simulink model "General_MG"  (R2024a)
settings: Solver=VariableStepAuto  StartTime=0.0  StopTime=10.0  RelTol=1e-3
values from neighbouring files (symbols this model uses):
  BarC = [Barc_11, Barc_12, Barc_13, Barc_14 ... (first row only)    [Global_Controller_Synthesis.m]    (also in globalControlDesign-Mohammad’s Laptop.m = zeros(numOfDGs * 3, numOfLines); globalControlDesign.m = zeros(numOfDGs * 3, numOfLines))
  C = [c_11,c_12,c_13,c_14 ... (first row only)    [Global_Controller_Synthesis.m]    (also in centralizedCodesignFeasibility.m = [statusL-ones(numOfDGs,1); statusG-1]; globalControlDesign-Mohammad’s Laptop.m = zeros(numOfLines, numOfDGs * 3); globalControlDesign.m = zeros(numOfLines, numOfDGs * 3))
  DG = cell(1, numOfDGs)    [evaluateDesigns.m]
  H = blkdiag(H, H_i)    [globalControlDesign-Mohammad’s Laptop.m]    (also in globalControlDesign.m)
  K = cell(1, numDGs)    [Centralized_Controller_For_DG.m]    (also in Centralized_Controller_For_DG_with_Constraints.m; ComputePassivityForDGs.m = sdpvar(1, 3, 'full'); GetPassivityForDGs.m = sdpvar(1, 3, 'full'); Global_Controller_Synthesis.m = cell(N, N))
  Line = cell(1, numOfLines)    [evaluateDesigns.m]
  numOfDGs = size(B_il,1)    [OptimizeMGparameters.m]    (also in OptimizepValsMethod1.m; centralizedCodesign.m; centralizedCodesignFeasibility.m; centralizedLocalControlDesign-Mohammad’s Laptop.m)
  numOfLines = size(B_il,2)    [OptimizeMGparameters.m]    (also in OptimizepValsMethod1.m; centralizedCodesign.m; centralizedCodesignFeasibility.m; centralizedLocalControlDesign-Mohammad’s Laptop.m)
  V_ref = 48    [Global_Controller_Synthesis.m]
settings Model: Creator=najaf  LastModifiedBy=najaf

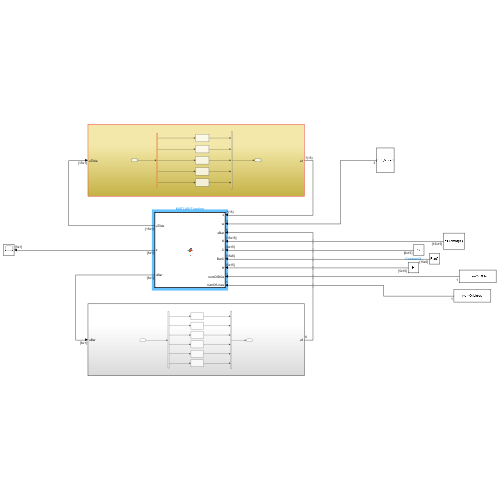
[thumbnail: Simulink's stored preview of the top-level diagram]
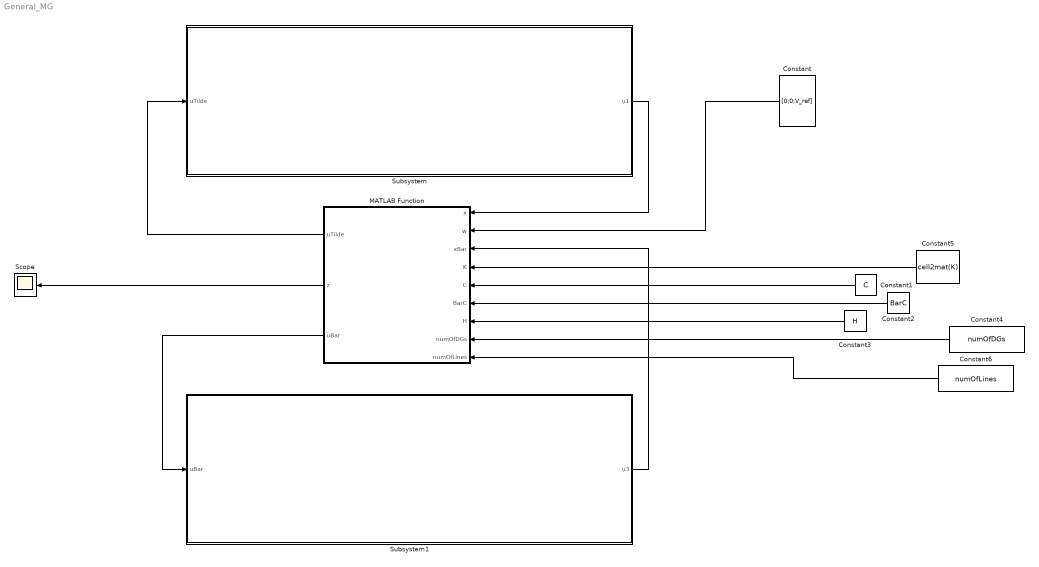
== system General_MG ==
  Constant : Constant  Value=[0;0;V_ref]
  Constant1 : Constant  Value=C
  Constant2 : Constant  Value=BarC
  Constant3 : Constant  Value=H
  Constant4 : Constant  Value=numOfDGs
  Constant5 : Constant  Value=cell2mat(K)
  Constant6 : Constant  Value=numOfLines
  MATLAB Function : MATLAB Function  TreatAsAtomicUnit=on
  Scope : Scope
  Subsystem : Subsystem
  Subsystem1 : Subsystem
  wires:
  Subsystem/1(u1) -> MATLAB Function/1(x)
  Subsystem1/1(u3) -> MATLAB Function/3(xBar)
  MATLAB Function/1(uTilde) -> Subsystem/1(uTilde)
  MATLAB Function/3(uBar) -> Subsystem1/1(uBar)
  MATLAB Function/2(z) -> Scope/1
  Constant/1 -> MATLAB Function/2(w)
  Constant1/1 -> MATLAB Function/5(C)
  Constant2/1 -> MATLAB Function/6(BarC)
  Constant3/1 -> MATLAB Function/7(H)
  Constant4/1 -> MATLAB Function/8(numOfDGs)
  Constant5/1 -> MATLAB Function/4(K)
  Constant6/1 -> MATLAB Function/9(numOfLines)

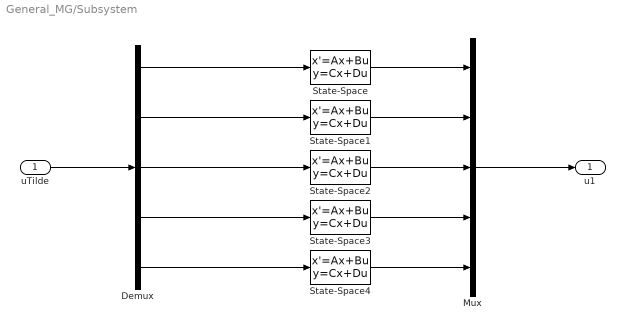
== system General_MG/Subsystem ==
  uTilde : Inport
  Demux : Demux  Outputs=5
  Mux : Mux  Inputs=5
  State-Space : StateSpace  A=DG{1}.A  B=DG{1}.B  C=eye(3)  D=zeros(3,1)  InitialCondition=0
  State-Space1 : StateSpace  A=DG{2}.A  B=DG{2}.B  C=eye(3)  D=zeros(3,1)  InitialCondition=0
  State-Space2 : StateSpace  A=DG{3}.A  B=DG{3}.B  C=eye(3)  D=zeros(3,1)  InitialCondition=0
  State-Space3 : StateSpace  A=DG{4}.A  B=DG{4}.B  C=eye(3)  D=zeros(3,1)  InitialCondition=0
  State-Space4 : StateSpace  A=DG{5}.A  B=DG{5}.B  C=eye(3)  D=zeros(3,1)  InitialCondition=0
  u1 : Outport
  wires:
  State-Space/1 -> Mux/1
  State-Space1/1 -> Mux/2
  State-Space2/1 -> Mux/3
  Mux/1 -> u1/1
  State-Space3/1 -> Mux/4
  State-Space4/1 -> Mux/5
  uTilde/1 -> Demux/1
  Demux/1 -> State-Space/1
  Demux/2 -> State-Space1/1
  Demux/3 -> State-Space2/1
  Demux/4 -> State-Space3/1
  Demux/5 -> State-Space4/1

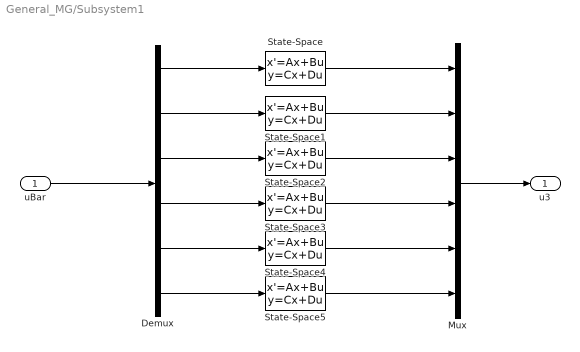
== system General_MG/Subsystem1 ==
  uBar : Inport
  Demux : Demux  Outputs=6
  Mux : Mux  Inputs=6
  State-Space : StateSpace  A=Line{1}.A  B=Line{1}.B  C=eye(1)  D=zeros(1)  InitialCondition=0
  State-Space1 : StateSpace  A=Line{2}.A  B=Line{2}.B  C=eye(1)  D=zeros(1)  InitialCondition=0
  State-Space2 : StateSpace  A=Line{3}.A  B=Line{3}.B  C=eye(1)  D=zeros(1)  InitialCondition=0
  State-Space3 : StateSpace  A=Line{4}.A  B=Line{4}.B  C=eye(1)  D=zeros(1)  InitialCondition=0
  State-Space4 : StateSpace  A=Line{5}.A  B=Line{5}.B  C=eye(1)  D=zeros(1)  InitialCondition=0
  State-Space5 : StateSpace  A=Line{6}.A  B=Line{6}.B  C=eye(1)  D=zeros(1)  InitialCondition=0
  u3 : Outport
  wires:
  Demux/1 -> State-Space/1
  Demux/2 -> State-Space1/1
  Demux/3 -> State-Space2/1
  Demux/4 -> State-Space3/1
  Demux/5 -> State-Space4/1
  Demux/6 -> State-Space5/1
  uBar/1 -> Demux/1
  State-Space/1 -> Mux/1
  State-Space1/1 -> Mux/2
  State-Space2/1 -> Mux/3
  State-Space3/1 -> Mux/4
  State-Space4/1 -> Mux/5
  State-Space5/1 -> Mux/6
  Mux/1 -> u3/1

== matlab function General_MG/MATLAB Function ==
  data: x input; uTilde output; w input; xBar input; K input; z output; uBar output; C input; BarC input; H input; numOfDGs input; numOfLines input
function [uTilde, z, uBar] = fcn(x, w, xBar, K, C, BarC, H, numOfDGs,numOfLines)
 % Define matrix operations
 uTilde = K*x + BarC*xBar + eye(3*numOfDGs)*w;
 uBar = C*x + zeros(numOfDGs,numOfLines)*xBar + zeros(numOfDGs,3*numOfDGs)*w;
 z = H*x + zeros(numOfDGs,numOfLines)*xBar + zeros(numOfDGs,3*numOfDGs)*w;
end
